simulink model "controls"  (R2022a)
settings: Solver=FixedStepDiscrete  StartTime=0.0  StopTime=30  FixedStep=dt  RelTol=1e-3
undefined symbols (not defined in the file or in its folder): R_z, R_z2, S_z, S_z2, T_z, T_z2
libraries: cstblocks x3
settings Model: Creator=phcs  LastModifiedBy=phcs

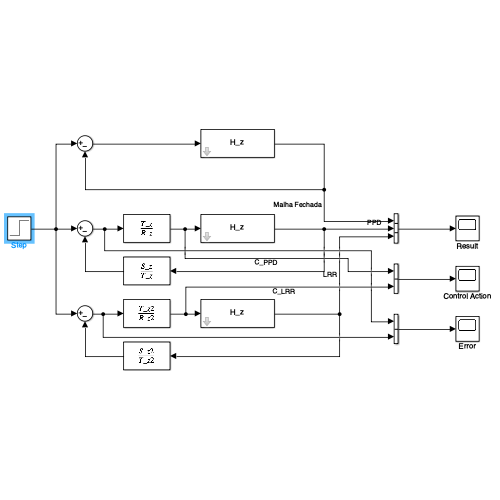
[thumbnail: Simulink's stored preview of the top-level diagram]
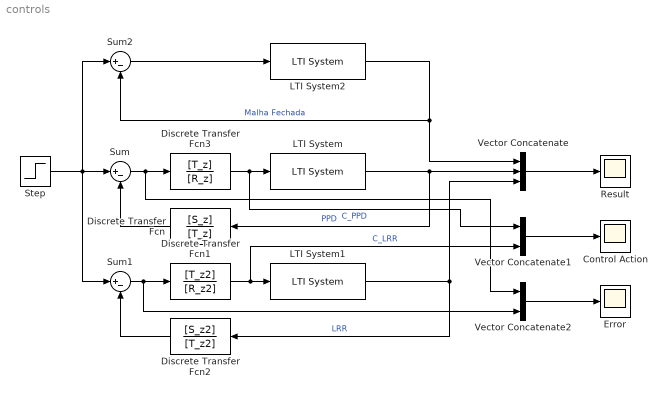
== system controls ==
  Control Action : Scope
  Discrete Transfer Fcn : DiscreteTransferFcn  Numerator=[S_z]  Denominator=[T_z]
  Discrete Transfer Fcn1 : DiscreteTransferFcn  Numerator=[T_z2]  Denominator=[R_z2]
  Discrete Transfer Fcn2 : DiscreteTransferFcn  Numerator=[S_z2]  Denominator=[T_z2]
  Discrete Transfer Fcn3 : DiscreteTransferFcn  Numerator=[T_z]  Denominator=[R_z]
  Error : Scope
  LTI System : cstblocks/LTI System  sys=H_z  IC=[]
  LTI System1 : cstblocks/LTI System  sys=H_z  IC=[]
  LTI System2 : cstblocks/LTI System  sys=H_z  IC=[]
  Result : Scope
  Step : Step  Time=0  SampleTime=0
  Sum : Sum  Inputs=|+-
  Sum1 : Sum  Inputs=|+-
  Sum2 : Sum  Inputs=|+-
  Vector Concatenate : Concatenate  NumInputs=3
  Vector Concatenate1 : Concatenate
  Vector Concatenate2 : Concatenate
  wires:
  Discrete Transfer Fcn3/1 -> Vector Concatenate1/1, LTI System/1  "C_PPD"
  Sum/1 -> Vector Concatenate2/1, Discrete Transfer Fcn3/1
  LTI System/1 -> Discrete Transfer Fcn/1, Vector Concatenate/2  "PPD"
  Discrete Transfer Fcn/1 -> Sum/2
  Vector Concatenate/1 -> Result/1
  Sum1/1 -> Vector Concatenate2/2, Discrete Transfer Fcn1/1
  LTI System1/1 -> Discrete Transfer Fcn2/1, Vector Concatenate/3  "LRR"
  Discrete Transfer Fcn2/1 -> Sum1/2
  Discrete Transfer Fcn1/1 -> LTI System1/1, Vector Concatenate1/2  "C_LRR"
  Step/1 -> Sum2/1, Sum1/1, Sum/1
  Vector Concatenate1/1 -> Control Action/1
  Sum2/1 -> LTI System2/1
  LTI System2/1 -> Vector Concatenate/1, Sum2/2  "Malha Fechada"
  Vector Concatenate2/1 -> Error/1
